simulink model "Mmc_GFL_template"  (R2024b)
settings: Solver=ode23t  StartTime=0.0  StopTime=.3  FixedStep=Ts_Power
undefined symbols (not defined in the file): Ch, Cm, Cmo, Fnom, fs, I_b, Ipp_b, kicir, kiout, kip, kpcir, kpout, kpp, L, L0, Nb_PM, R0, Rdis, Rh, Rm, SCR, SigmaM, Snom, Ts_Power, V_b, VDCm, VDCp, Vnom_AC, Vnom_PM, w_b, Zn
libraries: spsIGBTDiodeLib x48, spsSeriesRLCBranchLib x42, spsVoltageMeasurementLib x17, spsTriangleGeneratorLib x12, spsCurrentMeasurementLib x7, eePwmGeneratorMultilevel x7, slpidlib x6, spsFirstOrderFilterLib x4, spsabctodq0Lib x3, spsGroundLib x2, spsDCVoltageSourceLib x2, spsThreePhaseVIMeasurementLib x2
(part 3 of 3)

== matlab function Mmc_GFL_template/MMC/modulation/Sorting pb/MATLAB Function ==
  data: Usm input; N input; Ons_next output; Sigmam input; Iarm input; Ons input
function Ons_next = SmFiringSorting(Usm, N, Sigmam, Iarm, Ons)
    %%%
    % SmFiringSorting -- SM firing sorting. -- C.SI on 5th, Oct.
    %% Inputs:
    % Usm - capacitor voltage on each SM;
    % N - number of SMs that needed to fire up;
    % Sigmam [%] - Maximum allowed voltage unbalance rate;
    % Iarm - arm current;
    % Ons (boolean) - indicate those SM(s) who are in series with the
    % source in the last control period;
    %% Outputs:
    % Ons_now (boolean) - indicate those SM(s) who should be in series with 
    % the source in this control period;
    %%%
    
    % number of SMs
    Nb = length(Usm);
    % initialize the on-state boolean array
    Ons_next = zeros(Nb, 1); 
    % rank the SMs in the order of descendance
    [~, order] = sort(Usm, 'descend');
    
    if max(abs(1-Usm)) > Sigmam/100
        % Over the maximum unbalance acceptance
        if Iarm > 0
            % charge the capacitors with lowest voltages
            Ons_next(order(Nb-N+1: Nb)) = ~Ons_next(order(Nb-N+1: Nb));
        else
            % discharge the capacitors with highest voltages
            Ons_next(order(1: N)) = ~Ons_next(order(1: N));
        end

    else
        if N-sum(Ons) ==  0
            % if we don't need to change the number of SM that is on
            Ons_next = Ons;
        
        elseif N-sum(Ons) > 0
            % if we need more SMs are to be on-state

            % number of SMs that needed to be changed the state
            DeltaN = N-sum(Ons);
            % keep previously being on SMs still being on
            Ons_next = Ons;

            if Iarm > 0
                % charge the capacitors with lowest voltages
                for i = 1: Nb
                    if DeltaN <= 0
                        break;
                    end
                    % if the SM is off and still need more SM
                    if Ons(order(Nb-i+1)) == false
                        DeltaN = DeltaN - 1;
                        Ons_next(order(Nb-i+1)) = true;
                    end
                end

            else
                % discharge the capacitors with highest voltages
                for i = 1: Nb
                    if DeltaN <= 0
                        break;
                    end
                    % if the SM is off and still need more SM
                    if Ons(order(i)) == false
                        DeltaN = DeltaN - 1;
                        Ons_next(order(i)) = true;
                    end
                end
            end

        else
            % if we need less SMs are to be on-state

            % number of SMs that needed to be changed the state
            DeltaN = sum(Ons)-N;
            % keep previously being on SMs still being on
            Ons_next = Ons;

            if Iarm > 0
                % remove the capacitor with highest voltage
                for i = 1: Nb
                    if DeltaN <= 0
                        break;
                    end
                    % if the SM is on and still need less SM
                    if Ons(order(i)) == true
                        DeltaN = DeltaN - 1;
                        Ons_next(order(i)) = false;
                    end
                end

            else
                % remove the capacitor with lowest voltage
                for i = 1: Nb
                    if DeltaN <= 0
                        break;
                    end
                    % if the SM is on and still need less SM
                    if Ons(order(Nb-i+1)) == true
                        DeltaN = DeltaN - 1;
                        Ons_next(order(Nb-i+1)) = false;
                    end
                end
            end
        end
    end
end

== matlab function Mmc_GFL_template/MMC/modulation/Sorting pb/MATLAB Function1 ==
  data: u input; y output
function y = FiringSorting(u)
    y = u;
    for i = 1: length(u)
        if mod(i, 2) == 1
            y(i) = u(int16(i/2));
        else
            y(i) = u(int16(i/2+length(u)/2));
        end
    end
end

== matlab function Mmc_GFL_template/MMC/modulation/Sorting nb/MATLAB Function ==
  data: Usm input; N input; Ons_next output; Sigmam input; Iarm input; Ons input
function Ons_next = SmFiringSorting(Usm, N, Sigmam, Iarm, Ons)
    %%%
    % SmFiringSorting -- SM firing sorting. -- C.SI on 5th, Oct.
    %% Inputs:
    % Usm - capacitor voltage on each SM;
    % N - number of SMs that needed to fire up;
    % Sigmam [%] - Maximum allowed voltage unbalance rate;
    % Iarm - arm current;
    % Ons (boolean) - indicate those SM(s) who are in series with the
    % source in the last control period;
    %% Outputs:
    % Ons_now (boolean) - indicate those SM(s) who should be in series with 
    % the source in this control period;
    %%%
    
    % number of SMs
    Nb = length(Usm);
    % initialize the on-state boolean array
    Ons_next = zeros(Nb, 1); 
    % rank the SMs in the order of descendance
    [~, order] = sort(Usm, 'descend');
    
    if max(abs(1-Usm)) > Sigmam/100
        % Over the maximum unbalance acceptance
        if Iarm > 0
            % charge the capacitors with lowest voltages
            Ons_next(order(Nb-N+1: Nb)) = ~Ons_next(order(Nb-N+1: Nb));
        else
            % discharge the capacitors with highest voltages
            Ons_next(order(1: N)) = ~Ons_next(order(1: N));
        end

    else
        if N-sum(Ons) ==  0
            % if we don't need to change the number of SM that is on
            Ons_next = Ons;
        
        elseif N-sum(Ons) > 0
            % if we need more SMs are to be on-state

            % number of SMs that needed to be changed the state
            DeltaN = N-sum(Ons);
            % keep previously being on SMs still being on
            Ons_next = Ons;

            if Iarm > 0
                % charge the capacitors with lowest voltages
                for i = 1: Nb
                    if DeltaN <= 0
                        break;
                    end
                    % if the SM is off and still need more SM
                    if Ons(order(Nb-i+1)) == false
                        DeltaN = DeltaN - 1;
                        Ons_next(order(Nb-i+1)) = true;
                    end
                end

            else
                % discharge the capacitors with highest voltages
                for i = 1: Nb
                    if DeltaN <= 0
                        break;
                    end
                    % if the SM is off and still need more SM
                    if Ons(order(i)) == false
                        DeltaN = DeltaN - 1;
                        Ons_next(order(i)) = true;
                    end
                end
            end

        else
            % if we need less SMs are to be on-state

            % number of SMs that needed to be changed the state
            DeltaN = sum(Ons)-N;
            % keep previously being on SMs still being on
            Ons_next = Ons;

            if Iarm > 0
                % remove the capacitor with highest voltage
                for i = 1: Nb
                    if DeltaN <= 0
                        break;
                    end
                    % if the SM is on and still need less SM
                    if Ons(order(i)) == true
                        DeltaN = DeltaN - 1;
                        Ons_next(order(i)) = false;
                    end
                end

            else
                % remove the capacitor with lowest voltage
                for i = 1: Nb
                    if DeltaN <= 0
                        break;
                    end
                    % if the SM is on and still need less SM
                    if Ons(order(Nb-i+1)) == true
                        DeltaN = DeltaN - 1;
                        Ons_next(order(Nb-i+1)) = false;
                    end
                end
            end
        end
    end
end

== matlab function Mmc_GFL_template/MMC/modulation/Sorting nb/MATLAB Function1 ==
  data: u input; y output
function y = FiringSorting(u)
    y = u;
    for i = 1: length(u)
        if mod(i, 2) == 1
            y(i) = u(int16(i/2));
        else
            y(i) = u(int16(i/2+length(u)/2));
        end
    end
end

== matlab function Mmc_GFL_template/MMC/modulation/Sorting pc/MATLAB Function ==
  data: Usm input; N input; Ons_next output; Sigmam input; Iarm input; Ons input
function Ons_next = SmFiringSorting(Usm, N, Sigmam, Iarm, Ons)
    %%%
    % SmFiringSorting -- SM firing sorting. -- C.SI on 5th, Oct.
    %% Inputs:
    % Usm - capacitor voltage on each SM;
    % N - number of SMs that needed to fire up;
    % Sigmam [%] - Maximum allowed voltage unbalance rate;
    % Iarm - arm current;
    % Ons (boolean) - indicate those SM(s) who are in series with the
    % source in the last control period;
    %% Outputs:
    % Ons_now (boolean) - indicate those SM(s) who should be in series with 
    % the source in this control period;
    %%%
    
    % number of SMs
    Nb = length(Usm);
    % initialize the on-state boolean array
    Ons_next = zeros(Nb, 1); 
    % rank the SMs in the order of descendance
    [~, order] = sort(Usm, 'descend');
    
    if max(abs(1-Usm)) > Sigmam/100
        % Over the maximum unbalance acceptance
        if Iarm > 0
            % charge the capacitors with lowest voltages
            Ons_next(order(Nb-N+1: Nb)) = ~Ons_next(order(Nb-N+1: Nb));
        else
            % discharge the capacitors with highest voltages
            Ons_next(order(1: N)) = ~Ons_next(order(1: N));
        end

    else
        if N-sum(Ons) ==  0
            % if we don't need to change the number of SM that is on
            Ons_next = Ons;
        
        elseif N-sum(Ons) > 0
            % if we need more SMs are to be on-state

            % number of SMs that needed to be changed the state
            DeltaN = N-sum(Ons);
            % keep previously being on SMs still being on
            Ons_next = Ons;

            if Iarm > 0
                % charge the capacitors with lowest voltages
                for i = 1: Nb
                    if DeltaN <= 0
                        break;
                    end
                    % if the SM is off and still need more SM
                    if Ons(order(Nb-i+1)) == false
                        DeltaN = DeltaN - 1;
                        Ons_next(order(Nb-i+1)) = true;
                    end
                end

            else
                % discharge the capacitors with highest voltages
                for i = 1: Nb
                    if DeltaN <= 0
                        break;
                    end
                    % if the SM is off and still need more SM
                    if Ons(order(i)) == false
                        DeltaN = DeltaN - 1;
                        Ons_next(order(i)) = true;
                    end
                end
            end

        else
            % if we need less SMs are to be on-state

            % number of SMs that needed to be changed the state
            DeltaN = sum(Ons)-N;
            % keep previously being on SMs still being on
            Ons_next = Ons;

            if Iarm > 0
                % remove the capacitor with highest voltage
                for i = 1: Nb
                    if DeltaN <= 0
                        break;
                    end
                    % if the SM is on and still need less SM
                    if Ons(order(i)) == true
                        DeltaN = DeltaN - 1;
                        Ons_next(order(i)) = false;
                    end
                end

            else
                % remove the capacitor with lowest voltage
                for i = 1: Nb
                    if DeltaN <= 0
                        break;
                    end
                    % if the SM is on and still need less SM
                    if Ons(order(Nb-i+1)) == true
                        DeltaN = DeltaN - 1;
                        Ons_next(order(Nb-i+1)) = false;
                    end
                end
            end
        end
    end
end

== matlab function Mmc_GFL_template/MMC/modulation/Sorting pc/MATLAB Function1 ==
  data: u input; y output
function y = FiringSorting(u)
    y = u;
    for i = 1: length(u)
        if mod(i, 2) == 1
            y(i) = u(int16(i/2));
        else
            y(i) = u(int16(i/2+length(u)/2));
        end
    end
end

== matlab function Mmc_GFL_template/MMC/modulation/Sorting nc/MATLAB Function ==
  data: Usm input; N input; Ons_next output; Sigmam input; Iarm input; Ons input
function Ons_next = SmFiringSorting(Usm, N, Sigmam, Iarm, Ons)
    %%%
    % SmFiringSorting -- SM firing sorting. -- C.SI on 5th, Oct.
    %% Inputs:
    % Usm - capacitor voltage on each SM;
    % N - number of SMs that needed to fire up;
    % Sigmam [%] - Maximum allowed voltage unbalance rate;
    % Iarm - arm current;
    % Ons (boolean) - indicate those SM(s) who are in series with the
    % source in the last control period;
    %% Outputs:
    % Ons_now (boolean) - indicate those SM(s) who should be in series with 
    % the source in this control period;
    %%%
    
    % number of SMs
    Nb = length(Usm);
    % initialize the on-state boolean array
    Ons_next = zeros(Nb, 1); 
    % rank the SMs in the order of descendance
    [~, order] = sort(Usm, 'descend');
    
    if max(abs(1-Usm)) > Sigmam/100
        % Over the maximum unbalance acceptance
        if Iarm > 0
            % charge the capacitors with lowest voltages
            Ons_next(order(Nb-N+1: Nb)) = ~Ons_next(order(Nb-N+1: Nb));
        else
            % discharge the capacitors with highest voltages
            Ons_next(order(1: N)) = ~Ons_next(order(1: N));
        end

    else
        if N-sum(Ons) ==  0
            % if we don't need to change the number of SM that is on
            Ons_next = Ons;
        
        elseif N-sum(Ons) > 0
            % if we need more SMs are to be on-state

            % number of SMs that needed to be changed the state
            DeltaN = N-sum(Ons);
            % keep previously being on SMs still being on
            Ons_next = Ons;

            if Iarm > 0
                % charge the capacitors with lowest voltages
                for i = 1: Nb
                    if DeltaN <= 0
                        break;
                    end
                    % if the SM is off and still need more SM
                    if Ons(order(Nb-i+1)) == false
                        DeltaN = DeltaN - 1;
                        Ons_next(order(Nb-i+1)) = true;
                    end
                end

            else
                % discharge the capacitors with highest voltages
                for i = 1: Nb
                    if DeltaN <= 0
                        break;
                    end
                    % if the SM is off and still need more SM
                    if Ons(order(i)) == false
                        DeltaN = DeltaN - 1;
                        Ons_next(order(i)) = true;
                    end
                end
            end

        else
            % if we need less SMs are to be on-state

            % number of SMs that needed to be changed the state
            DeltaN = sum(Ons)-N;
            % keep previously being on SMs still being on
            Ons_next = Ons;

            if Iarm > 0
                % remove the capacitor with highest voltage
                for i = 1: Nb
                    if DeltaN <= 0
                        break;
                    end
                    % if the SM is on and still need less SM
                    if Ons(order(i)) == true
                        DeltaN = DeltaN - 1;
                        Ons_next(order(i)) = false;
                    end
                end

            else
                % remove the capacitor with lowest voltage
                for i = 1: Nb
                    if DeltaN <= 0
                        break;
                    end
                    % if the SM is on and still need less SM
                    if Ons(order(Nb-i+1)) == true
                        DeltaN = DeltaN - 1;
                        Ons_next(order(Nb-i+1)) = false;
                    end
                end
            end
        end
    end
end

== matlab function Mmc_GFL_template/MMC/modulation/Sorting nc/MATLAB Function1 ==
  data: u input; y output
function y = FiringSorting(u)
    y = u;
    for i = 1: length(u)
        if mod(i, 2) == 1
            y(i) = u(int16(i/2));
        else
            y(i) = u(int16(i/2+length(u)/2));
        end
    end
end

== matlab function Mmc_GFL_template/MMC/modulation/Sorting pb1/MATLAB Function1 ==
  data: u input; y output
function y = FiringSorting(u)
    y = u;
    for i = 1: length(u)
        if mod(i, 2) == 1
            y(i) = u(int16(i/2));
        else
            y(i) = u(int16(i/2+length(u)/2));
        end
    end
end

== matlab function Mmc_GFL_template/MMC/modulation/Subsystem1/Upper arm a ==
  data: signals input; n_pwm output
function n_pwm = PWM(signals)
% Name: PWM
% Input: the PWM gate signal of one arm.
%        40 signals with 0 or 1 
% Output: the number of activated submodels in one arm
%         0<Int(n_pwm)<20
% Discription: Get the number of activated submodels from the PWM gate
% signals

    % Identify if there is 40 signal inputs
    if length(signals) ~= 8
        error('Input must be a vector with exactly 40 elements.');
    end
    % Select the odd signal (the gate signal for upper side switch)
    %Sig_up = signals(1:2:end);
    counter = 0;
    if signals(1)==1 && signals(3)==1
        counter = counter + 1;
    end
    if signals(2)==1 && signals(4)==1
        counter = counter + 1;
    end
    if signals(5)==1 && signals(7)==1
        counter = counter + 1;
    end
    if signals(6)==1 && signals(8)==1
        counter = counter + 1;
    end

    % Count how many submodel is activated
    n_pwm = 2 - counter;%2 - sum(Sig_up);
    %counter = 0;
end

== matlab function Mmc_GFL_template/MMC/modulation/Subsystem7/Upper arm a ==
  data: signals input; n_pwm output
function n_pwm = PWM(signals)
% Name: PWM
% Input: the PWM gate signal of one arm.
%        40 signals with 0 or 1 
% Output: the number of activated submodels in one arm
%         0<Int(n_pwm)<20
% Discription: Get the number of activated submodels from the PWM gate
% signals

    % Identify if there is 40 signal inputs
    if length(signals) ~= 8
        error('Input must be a vector with exactly 40 elements.');
    end
    % Select the odd signal (the gate signal for upper side switch)
    %Sig_up = signals(1:2:end);
    counter = 0;
    if signals(1)==1 && signals(3)==1
        counter = counter + 1;
    end
    if signals(2)==1 && signals(4)==1
        counter = counter + 1;
    end
    if signals(5)==1 && signals(7)==1
        counter = counter + 1;
    end
    if signals(6)==1 && signals(8)==1
        counter = counter + 1;
    end

    % Count how many submodel is activated
    n_pwm = 2 - counter;%2 - sum(Sig_up);
    %counter = 0;
end

== matlab function Mmc_GFL_template/MMC/modulation/Subsystem8/Upper arm a ==
  data: signals input; n_pwm output
function n_pwm = PWM(signals)
% Name: PWM
% Input: the PWM gate signal of one arm.
%        40 signals with 0 or 1 
% Output: the number of activated submodels in one arm
%         0<Int(n_pwm)<20
% Discription: Get the number of activated submodels from the PWM gate
% signals

    % Identify if there is 40 signal inputs
    if length(signals) ~= 8
        error('Input must be a vector with exactly 40 elements.');
    end
    % Select the odd signal (the gate signal for upper side switch)
    %Sig_up = signals(1:2:end);
    counter = 0;
    if signals(1)==1 && signals(3)==1
        counter = counter + 1;
    end
    if signals(2)==1 && signals(4)==1
        counter = counter + 1;
    end
    if signals(5)==1 && signals(7)==1
        counter = counter + 1;
    end
    if signals(6)==1 && signals(8)==1
        counter = counter + 1;
    end

    % Count how many submodel is activated
    n_pwm = 2 - counter;%2 - sum(Sig_up);
    %counter = 0;
end

== matlab function Mmc_GFL_template/MMC/modulation/Subsystem10/Upper arm a ==
  data: signals input; n_pwm output
function n_pwm = PWM(signals)
% Name: PWM
% Input: the PWM gate signal of one arm.
%        40 signals with 0 or 1 
% Output: the number of activated submodels in one arm
%         0<Int(n_pwm)<20
% Discription: Get the number of activated submodels from the PWM gate
% signals

    % Identify if there is 40 signal inputs
    if length(signals) ~= 8
        error('Input must be a vector with exactly 40 elements.');
    end
    % Select the odd signal (the gate signal for upper side switch)
    %Sig_up = signals(1:2:end);
    counter = 0;
    if signals(1)==1 && signals(3)==1
        counter = counter + 1;
    end
    if signals(2)==1 && signals(4)==1
        counter = counter + 1;
    end
    if signals(5)==1 && signals(7)==1
        counter = counter + 1;
    end
    if signals(6)==1 && signals(8)==1
        counter = counter + 1;
    end

    % Count how many submodel is activated
    n_pwm = 2 - counter;%2 - sum(Sig_up);
    %counter = 0;
end

== matlab function Mmc_GFL_template/MMC/modulation/Sorting pa/MATLAB Function ==
  data: Usm input; N input; Ons_next output; Sigmam input; Iarm input; Ons input
function Ons_next = SmFiringSorting(Usm, N, Sigmam, Iarm, Ons)
    %%%
    % SmFiringSorting -- SM firing sorting. -- C.SI on 5th, Oct.
    %% Inputs:
    % Usm - capacitor voltage on each SM;
    % N - number of SMs that needed to fire up;
    % Sigmam [%] - Maximum allowed voltage unbalance rate;
    % Iarm - arm current;
    % Ons (boolean) - indicate those SM(s) who are in series with the
    % source in the last control period;
    %% Outputs:
    % Ons_now (boolean) - indicate those SM(s) who should be in series with 
    % the source in this control period;
    %%%
    
    % number of SMs
    Nb = length(Usm);
    % initialize the on-state boolean array
    Ons_next = zeros(Nb, 1); 
    % rank the SMs in the order of descendance
    [~, order] = sort(Usm, 'descend');
    
    if max(abs(1-Usm)) > Sigmam/100
        % Over the maximum unbalance acceptance
        if Iarm > 0
            % charge the capacitors with lowest voltages
            Ons_next(order(Nb-N+1: Nb)) = ~Ons_next(order(Nb-N+1: Nb));
        else
            % discharge the capacitors with highest voltages
            Ons_next(order(1: N)) = ~Ons_next(order(1: N));
        end

    else
        if N-sum(Ons) ==  0
            % if we don't need to change the number of SM that is on
            Ons_next = Ons;
        
        elseif N-sum(Ons) > 0
            % if we need more SMs are to be on-state

            % number of SMs that needed to be changed the state
            DeltaN = N-sum(Ons);
            % keep previously being on SMs still being on
            Ons_next = Ons;

            if Iarm > 0
                % charge the capacitors with lowest voltages
                for i = 1: Nb
                    if DeltaN <= 0
                        break;
                    end
                    % if the SM is off and still need more SM
                    if Ons(order(Nb-i+1)) == false
                        DeltaN = DeltaN - 1;
                        Ons_next(order(Nb-i+1)) = true;
                    end
                end

            else
                % discharge the capacitors with highest voltages
                for i = 1: Nb
                    if DeltaN <= 0
                        break;
                    end
                    % if the SM is off and still need more SM
                    if Ons(order(i)) == false
                        DeltaN = DeltaN - 1;
                        Ons_next(order(i)) = true;
                    end
                end
            end

        else
            % if we need less SMs are to be on-state

            % number of SMs that needed to be changed the state
            DeltaN = sum(Ons)-N;
            % keep previously being on SMs still being on
            Ons_next = Ons;

            if Iarm > 0
                % remove the capacitor with highest voltage
                for i = 1: Nb
                    if DeltaN <= 0
                        break;
                    end
                    % if the SM is on and still need less SM
                    if Ons(order(i)) == true
                        DeltaN = DeltaN - 1;
                        Ons_next(order(i)) = false;
                    end
                end

            else
                % remove the capacitor with lowest voltage
                for i = 1: Nb
                    if DeltaN <= 0
                        break;
                    end
                    % if the SM is on and still need less SM
                    if Ons(order(Nb-i+1)) == true
                        DeltaN = DeltaN - 1;
                        Ons_next(order(Nb-i+1)) = false;
                    end
                end
            end
        end
    end
end

== matlab function Mmc_GFL_template/MMC/modulation/Sorting pa/MATLAB Function1 ==
  data: u input; y output
function y = FiringSorting(u)
    y = u;
    for i = 1: length(u)
        if mod(i, 2) == 1
            y(i) = u(int16(i/2));
        else
            y(i) = u(int16(i/2+length(u)/2));
        end
    end
end

== matlab function Mmc_GFL_template/MMC/modulation/Subsystem9/Upper arm a ==
  data: signals input; n_pwm output
function n_pwm = PWM(signals)
% Name: PWM
% Input: the PWM gate signal of one arm.
%        40 signals with 0 or 1 
% Output: the number of activated submodels in one arm
%         0<Int(n_pwm)<20
% Discription: Get the number of activated submodels from the PWM gate
% signals

    % Identify if there is 40 signal inputs
    if length(signals) ~= 8
        error('Input must be a vector with exactly 40 elements.');
    end
    % Select the odd signal (the gate signal for upper side switch)
    %Sig_up = signals(1:2:end);
    counter = 0;
    if signals(1)==1 && signals(3)==1
        counter = counter + 1;
    end
    if signals(2)==1 && signals(4)==1
        counter = counter + 1;
    end
    if signals(5)==1 && signals(7)==1
        counter = counter + 1;
    end
    if signals(6)==1 && signals(8)==1
        counter = counter + 1;
    end

    % Count how many submodel is activated
    n_pwm = 2 - counter;%2 - sum(Sig_up);
    %counter = 0;
end

== matlab function Mmc_GFL_template/MMC/modulation/Subsystem11/Upper arm a ==
  data: signals input; n_pwm output
function n_pwm = PWM(signals)
% Name: PWM
% Input: the PWM gate signal of one arm.
%        40 signals with 0 or 1 
% Output: the number of activated submodels in one arm
%         0<Int(n_pwm)<20
% Discription: Get the number of activated submodels from the PWM gate
% signals

    % Identify if there is 40 signal inputs
    if length(signals) ~= 8
        error('Input must be a vector with exactly 40 elements.');
    end
    % Select the odd signal (the gate signal for upper side switch)
    %Sig_up = signals(1:2:end);
    counter = 0;
    if signals(1)==1 && signals(3)==1
        counter = counter + 1;
    end
    if signals(2)==1 && signals(4)==1
        counter = counter + 1;
    end
    if signals(5)==1 && signals(7)==1
        counter = counter + 1;
    end
    if signals(6)==1 && signals(8)==1
        counter = counter + 1;
    end

    % Count how many submodel is activated
    n_pwm = 2 - counter;%2 - sum(Sig_up);
    %counter = 0;
end

== matlab function Mmc_GFL_template/MMC/modulation/Subsystem6/Upper arm a ==
  data: signals input; n_pwm output
function n_pwm = PWM(signals)
% Name: PWM
% Input: the PWM gate signal of one arm.
%        40 signals with 0 or 1 
% Output: the number of activated submodels in one arm
%         0<Int(n_pwm)<20
% Discription: Get the number of activated submodels from the PWM gate
% signals

    % Identify if there is 40 signal inputs
    if length(signals) ~= 4
        error('Input must be a vector with exactly 40 elements.');
    end
    % Select the odd signal (the gate signal for upper side switch)
    Sig_up = signals(1:2:end);
    % Count how many submodel is activated
    n_pwm = 2 - sum(Sig_up);
end

== matlab function Mmc_GFL_template/MMC/modulation/Sorting na/MATLAB Function ==
  data: Usm input; N input; Ons_next output; Sigmam input; Iarm input; Ons input
function Ons_next = SmFiringSorting(Usm, N, Sigmam, Iarm, Ons)
    %%%
    % SmFiringSorting -- SM firing sorting. -- C.SI on 5th, Oct.
    %% Inputs:
    % Usm - capacitor voltage on each SM;
    % N - number of SMs that needed to fire up;
    % Sigmam [%] - Maximum allowed voltage unbalance rate;
    % Iarm - arm current;
    % Ons (boolean) - indicate those SM(s) who are in series with the
    % source in the last control period;
    %% Outputs:
    % Ons_now (boolean) - indicate those SM(s) who should be in series with 
    % the source in this control period;
    %%%
    
    % number of SMs
    Nb = length(Usm);
    % initialize the on-state boolean array
    Ons_next = zeros(Nb, 1); 
    % rank the SMs in the order of descendance
    [~, order] = sort(Usm, 'descend');
    
    if max(abs(1-Usm)) > Sigmam/100
        % Over the maximum unbalance acceptance
        if Iarm > 0
            % charge the capacitors with lowest voltages
            Ons_next(order(Nb-N+1: Nb)) = ~Ons_next(order(Nb-N+1: Nb));
        else
            % discharge the capacitors with highest voltages
            Ons_next(order(1: N)) = ~Ons_next(order(1: N));
        end

    else
        if N-sum(Ons) ==  0
            % if we don't need to change the number of SM that is on
            Ons_next = Ons;
        
        elseif N-sum(Ons) > 0
            % if we need more SMs are to be on-state

            % number of SMs that needed to be changed the state
            DeltaN = N-sum(Ons);
            % keep previously being on SMs still being on
            Ons_next = Ons;

            if Iarm > 0
                % charge the capacitors with lowest voltages
                for i = 1: Nb
                    if DeltaN <= 0
                        break;
                    end
                    % if the SM is off and still need more SM
                    if Ons(order(Nb-i+1)) == false
                        DeltaN = DeltaN - 1;
                        Ons_next(order(Nb-i+1)) = true;
                    end
                end

            else
                % discharge the capacitors with highest voltages
                for i = 1: Nb
                    if DeltaN <= 0
                        break;
                    end
                    % if the SM is off and still need more SM
                    if Ons(order(i)) == false
                        DeltaN = DeltaN - 1;
                        Ons_next(order(i)) = true;
                    end
                end
            end

        else
            % if we need less SMs are to be on-state

            % number of SMs that needed to be changed the state
            DeltaN = sum(Ons)-N;
            % keep previously being on SMs still being on
            Ons_next = Ons;

            if Iarm > 0
                % remove the capacitor with highest voltage
                for i = 1: Nb
                    if DeltaN <= 0
                        break;
                    end
                    % if the SM is on and still need less SM
                    if Ons(order(i)) == true
                        DeltaN = DeltaN - 1;
                        Ons_next(order(i)) = false;
                    end
                end

            else
                % remove the capacitor with lowest voltage
                for i = 1: Nb
                    if DeltaN <= 0
                        break;
                    end
                    % if the SM is on and still need less SM
                    if Ons(order(Nb-i+1)) == true
                        DeltaN = DeltaN - 1;
                        Ons_next(order(Nb-i+1)) = false;
                    end
                end
            end
        end
    end
end
